simulink model "ofdm_fdm"  (Simulink 5.0)
settings: Solver=ode45  StartTime=0.0  StopTime=1  RelTol=1e-3
undefined symbols (not defined in the file): Fs
libraries: dspsrcs4 x10, dspsigops x6, commdigbbndpm2 x5, commrandsrc2 x5, dsparch4 x5, dspsnks4 x2, dspbuff3 x2, dspxfrm3 x1
settings Model: LastModifiedBy=Daiming Qu

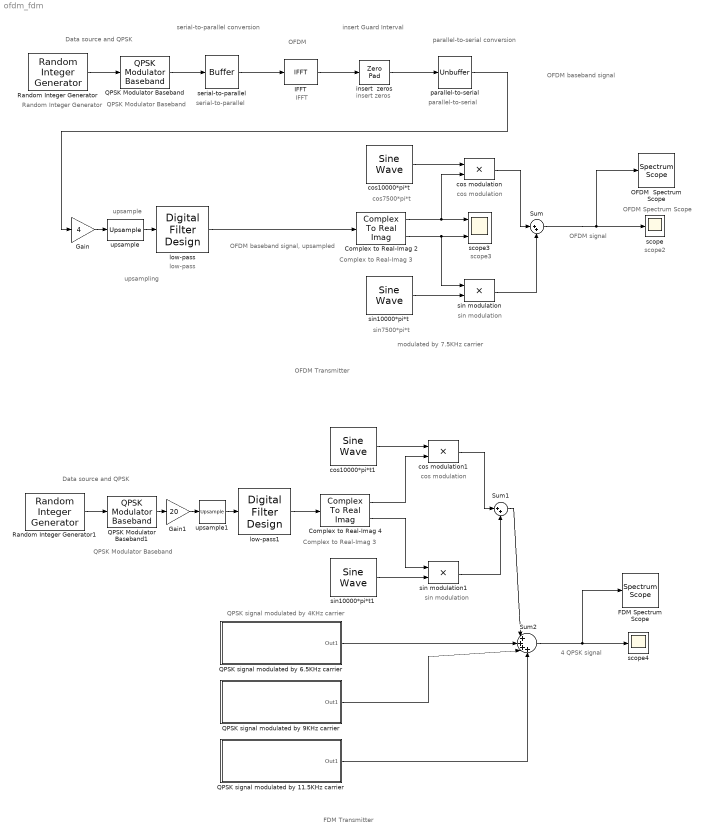
== system ofdm_fdm ==
  note: cos modulation
  note: Complex to
      | Real-Imag
      | 3
  note: Data source and QPSK
  note: QPSK
      | Modulator
      | Baseband
  note: QPSK signal modulated by 4KHz carrier
  note: sin modulation
  note: 4 QPSK signal
  note: FDM Transmitter
  note: serial-to-parallel
      |  conversion
  note: parallel-to-serial
      | conversion
  note: insert
      | Guard Interval
  note: OFDM
  note: modulated by
      | 7.5KHz carrier
  note: OFDM signal
  note: Random Integer
      | Generator
  note: QPSK
      | Modulator
      | Baseband
  note: serial-to-parallel
  note: IFFT
  note: insert
      | zeros
  note: parallel-to-serial
  note: upsample
  note: low-pass
  note: Complex to
      | Real-Imag
      | 3
  note: cos modulation
  note: sin modulation
  note: cos7500*pi*t
  note: sin7500*pi*t
  note: scope2
  note: OFDM Spectrum
      | Scope
  note: OFDM baseband signal
  note: scope3
  note: OFDM baseband
      | signal, upsampled
  note: upsampling
  note: Data source and QPSK
  note: OFDM Transmitter
  Complex to Real-Imag 2 : ComplexToRealImag
  Complex to Real-Imag 4 : ComplexToRealImag
  FDM Spectrum Scope : dspsnks4/Spectrum Scope  ScopeProperties=on  Domain=Frequency  HorizSpan=1  UseBuffer=on  BufferSize=2048  Overlap=0  inpFftLenInherit=off  FFTlength=2048  numAvg=128  DisplayProperties=off  AxisGrid=on  Memory=off  FrameNumber=on  AxisLegend=off  AxisZoom=off  OpenScopeAtSimStart=on  OpenScopeImmediately=off  FigPos=[34 274 560 420]  AxisProperties=off  XUnits=Hertz  XRange=[-Fs/2...Fs/2]  InheritXIncr=on  XIncr=1.0  XLabel=Samples  YUnits=dB  YLabel=Magnitude, dB  LineProperties=off  LineColors=[0 0 1]
      settings: YMin=-65  YMax=5
  Gain : Gain  Gain=4  SaturateOnIntegerOverflow=on
  Gain1 : Gain  Gain=20  SaturateOnIntegerOverflow=on
  IFFT : dspxfrm3/IFFT  CompMethod=Trigonometric fcn  TableOpt=Speed  BitRevOrder=off  cs_in=off  SkipNorm=on  mode=Real
  OFDM  Spectrum Scope : dspsnks4/Spectrum Scope  ScopeProperties=on  Domain=Frequency  HorizSpan=1  UseBuffer=on  BufferSize=2048  Overlap=0  inpFftLenInherit=off  FFTlength=2048  numAvg=128  DisplayProperties=off  AxisGrid=on  Memory=off  FrameNumber=on  AxisLegend=off  AxisZoom=off  OpenScopeAtSimStart=on  OpenScopeImmediately=off  FigPos=[446 60 560 420]  AxisProperties=off  XUnits=Hertz  XRange=[-Fs/2...Fs/2]  InheritXIncr=on  XIncr=1.0  XLabel=Samples  YUnits=dB  YLabel=Magnitude, dB  LineProperties=off  LineColors=[0 0 1]
      settings: YMin=-45  YMax=15
  QPSK Modulator Baseband : commdigbbndpm2/QPSK Modulator Baseband  InType=Integer  Enc=Binary  Ph=0  numSamp=1
  QPSK Modulator Baseband1 : commdigbbndpm2/QPSK Modulator Baseband  InType=Integer  Enc=Binary  Ph=0  numSamp=1
  QPSK signal modulated by 11.5KHz carrier : Subsystem
  QPSK signal modulated by 6.5KHz carrier : Subsystem
  QPSK signal modulated by 9KHz carrier : Subsystem
  Random Integer Generator : commrandsrc2/Random Integer Generator  mul=4  seed=37  Ts=1/6400  frameBased=off  sampPerFrame=1  orient=off
  Random Integer Generator1 : commrandsrc2/Random Integer Generator  mul=4  seed=37  Ts=1/1600  frameBased=off  sampPerFrame=1  orient=off
  Sum : Sum  Inputs=|++  SaturateOnIntegerOverflow=on
  Sum1 : Sum  Inputs=|++  SaturateOnIntegerOverflow=on
  Sum2 : Sum  Inputs=|++++  SaturateOnIntegerOverflow=on
  cos modulation : Product  SaturateOnIntegerOverflow=on
  cos modulation1 : Product  SaturateOnIntegerOverflow=on
  cos10000*pi*t : dspsrcs4/Sine Wave  Amplitude=1  Frequency=7500  Phase=pi/2  SampleMode=Discrete  OutComplex=Real  CompMethod=Trigonometric fcn  TableSize=Speed  SampleTime=1/32000  SamplesPerFrame=1  dataType=double  wordLen=16  udDataType=sfix(16)  fracBitsMode=Best precision  numFracBits=14  ResetState=Restart at time zero
  cos10000*pi*t1 : dspsrcs4/Sine Wave  Amplitude=1  Frequency=4000  Phase=pi/2  SampleMode=Discrete  OutComplex=Real  CompMethod=Trigonometric fcn  TableSize=Speed  SampleTime=1/32000  SamplesPerFrame=1  dataType=double  wordLen=16  udDataType=sfix(16)  fracBitsMode=Best precision  numFracBits=14  ResetState=Restart at time zero
  insert  zeros : dspsigops/Zero Pad  padSigAt=End  zpadAlong=Columns  padNumOutRowsSpecMethod=User-specified  numOutRows=80  padNumOutColsSpecMethod=User-specified  numOutCols=1  trunc_flag=None
  low-pass : dsparch4/Digital Filter Design
  low-pass1 : dsparch4/Digital Filter Design
  parallel-to-serial : dspbuff3/Unbuffer  ic=0
  scope : Scope
      settings: YMin=-0.1  YMax=0.3  SaveName=ScopeData3
  scope3 : Scope  NumInputPorts=2
      settings: YMin=-0.1~-5  YMax=0.3~5
  scope4 : Scope
      settings: YMin=-0.1  YMax=0.3
  serial-to-parallel : dspbuff3/Buffer  N=64  V=0  ic=0
  sin modulation : Product  SaturateOnIntegerOverflow=on
  sin modulation1 : Product  SaturateOnIntegerOverflow=on
  sin10000*pi*t : dspsrcs4/Sine Wave  Amplitude=1  Frequency=7500  Phase=0  SampleMode=Discrete  OutComplex=Real  CompMethod=Trigonometric fcn  TableSize=Speed  SampleTime=1/32000  SamplesPerFrame=1  dataType=double  wordLen=16  udDataType=sfix(16)  fracBitsMode=Best precision  numFracBits=14  ResetState=Restart at time zero
  sin10000*pi*t1 : dspsrcs4/Sine Wave  Amplitude=1  Frequency=4000  Phase=0  SampleMode=Discrete  OutComplex=Real  CompMethod=Trigonometric fcn  TableSize=Speed  SampleTime=1/32000  SamplesPerFrame=1  dataType=double  wordLen=16  udDataType=sfix(16)  fracBitsMode=Best precision  numFracBits=14  ResetState=Restart at time zero
  upsample : dspsigops/Upsample  N=4  phase=1  ic=0  mode=Maintain input frame size
  upsample1 : dspsigops/Upsample  N=20  phase=1  ic=0  mode=Maintain input frame size
  wires:
  low-pass1/1 -> Complex to Real-Imag 4/1
  upsample1/1 -> low-pass1/1
  cos10000*pi*t1/1 -> cos modulation1/1
  sin modulation1/1 -> Sum1/2
  cos modulation1/1 -> Sum1/1
  Complex to Real-Imag 4/2 -> sin modulation1/1
  sin10000*pi*t1/1 -> sin modulation1/2
  Complex to Real-Imag 4/1 -> cos modulation1/2
  Random Integer Generator1/1 -> QPSK Modulator Baseband1/1
  Sum1/1 -> Sum2/1
  QPSK signal modulated by 11.5KHz carrier/1(Out1) -> Sum2/4
  Sum2/1 -> FDM Spectrum Scope/1, scope4/1
  QPSK signal modulated by 6.5KHz carrier/1(Out1) -> Sum2/2
  QPSK signal modulated by 9KHz carrier/1(Out1) -> Sum2/3
  insert  zeros/1 -> parallel-to-serial/1
  low-pass/1 -> Complex to Real-Imag 2/1
  cos10000*pi*t/1 -> cos modulation/1
  Complex to Real-Imag 2/1 -> cos modulation/2, scope3/1
  sin10000*pi*t/1 -> sin modulation/2
  Complex to Real-Imag 2/2 -> sin modulation/1, scope3/2
  cos modulation/1 -> Sum/1
  sin modulation/1 -> Sum/2
  Sum/1 -> scope/1, OFDM  Spectrum Scope/1
  serial-to-parallel/1 -> IFFT/1
  IFFT/1 -> insert  zeros/1
  Random Integer Generator/1 -> QPSK Modulator Baseband/1
  QPSK Modulator Baseband/1 -> serial-to-parallel/1
  upsample/1 -> low-pass/1
  parallel-to-serial/1 -> Gain/1
  Gain/1 -> upsample/1
  QPSK Modulator Baseband1/1 -> Gain1/1
  Gain1/1 -> upsample1/1

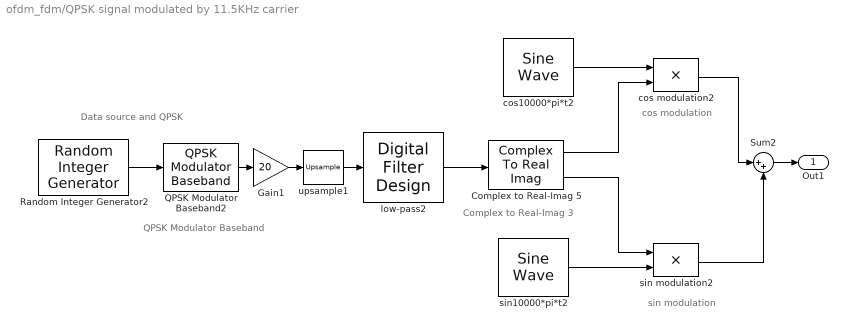
== system ofdm_fdm/QPSK signal modulated by 11.5KHz carrier ==
  note: cos modulation
  note: Complex to
      | Real-Imag
      | 3
  note: Data source and QPSK
  note: QPSK
      | Modulator
      | Baseband
  note: sin modulation
  Complex to Real-Imag 5 : ComplexToRealImag
  Gain1 : Gain  Gain=20  SaturateOnIntegerOverflow=on
  QPSK Modulator Baseband2 : commdigbbndpm2/QPSK Modulator Baseband  InType=Integer  Enc=Binary  Ph=0  numSamp=1
  Random Integer Generator2 : commrandsrc2/Random Integer Generator  mul=4  seed=15  Ts=1/1600  frameBased=off  sampPerFrame=1  orient=off
  Sum2 : Sum  Inputs=|++  SaturateOnIntegerOverflow=on
  cos modulation2 : Product  SaturateOnIntegerOverflow=on
  cos10000*pi*t2 : dspsrcs4/Sine Wave  Amplitude=1  Frequency=11500  Phase=pi/2  SampleMode=Discrete  OutComplex=Real  CompMethod=Trigonometric fcn  TableSize=Speed  SampleTime=1/32000  SamplesPerFrame=1  dataType=double  wordLen=16  udDataType=sfix(16)  fracBitsMode=Best precision  numFracBits=14  ResetState=Restart at time zero
  low-pass2 : dsparch4/Digital Filter Design
  sin modulation2 : Product  SaturateOnIntegerOverflow=on
  sin10000*pi*t2 : dspsrcs4/Sine Wave  Amplitude=1  Frequency=11500  Phase=0  SampleMode=Discrete  OutComplex=Real  CompMethod=Trigonometric fcn  TableSize=Speed  SampleTime=1/32000  SamplesPerFrame=1  dataType=double  wordLen=16  udDataType=sfix(16)  fracBitsMode=Best precision  numFracBits=14  ResetState=Restart at time zero
  upsample1 : dspsigops/Upsample  N=20  phase=1  ic=0  mode=Maintain input frame size
  Out1 : Outport
  wires:
  low-pass2/1 -> Complex to Real-Imag 5/1
  cos10000*pi*t2/1 -> cos modulation2/1
  sin modulation2/1 -> Sum2/2
  cos modulation2/1 -> Sum2/1
  Complex to Real-Imag 5/2 -> sin modulation2/1
  sin10000*pi*t2/1 -> sin modulation2/2
  Complex to Real-Imag 5/1 -> cos modulation2/2
  Random Integer Generator2/1 -> QPSK Modulator Baseband2/1
  Sum2/1 -> Out1/1
  Gain1/1 -> upsample1/1
  QPSK Modulator Baseband2/1 -> Gain1/1
  upsample1/1 -> low-pass2/1

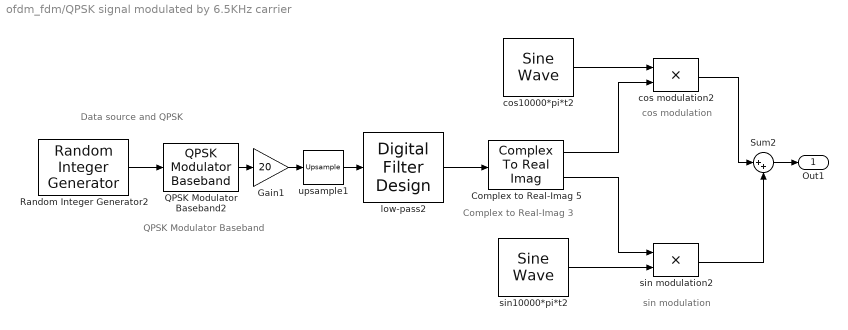
== system ofdm_fdm/QPSK signal modulated by 6.5KHz carrier ==
  note: cos modulation
  note: Complex to
      | Real-Imag
      | 3
  note: Data source and QPSK
  note: QPSK
      | Modulator
      | Baseband
  note: sin modulation
  Complex to Real-Imag 5 : ComplexToRealImag
  Gain1 : Gain  Gain=20  SaturateOnIntegerOverflow=on
  QPSK Modulator Baseband2 : commdigbbndpm2/QPSK Modulator Baseband  InType=Integer  Enc=Binary  Ph=0  numSamp=1
  Random Integer Generator2 : commrandsrc2/Random Integer Generator  mul=4  seed=76  Ts=1/1600  frameBased=off  sampPerFrame=1  orient=off
  Sum2 : Sum  Inputs=|++  SaturateOnIntegerOverflow=on
  cos modulation2 : Product  SaturateOnIntegerOverflow=on
  cos10000*pi*t2 : dspsrcs4/Sine Wave  Amplitude=1  Frequency=6500  Phase=pi/2  SampleMode=Discrete  OutComplex=Real  CompMethod=Trigonometric fcn  TableSize=Speed  SampleTime=1/32000  SamplesPerFrame=1  dataType=double  wordLen=16  udDataType=sfix(16)  fracBitsMode=Best precision  numFracBits=14  ResetState=Restart at time zero
  low-pass2 : dsparch4/Digital Filter Design
  sin modulation2 : Product  SaturateOnIntegerOverflow=on
  sin10000*pi*t2 : dspsrcs4/Sine Wave  Amplitude=1  Frequency=6500  Phase=0  SampleMode=Discrete  OutComplex=Real  CompMethod=Trigonometric fcn  TableSize=Speed  SampleTime=1/32000  SamplesPerFrame=1  dataType=double  wordLen=16  udDataType=sfix(16)  fracBitsMode=Best precision  numFracBits=14  ResetState=Restart at time zero
  upsample1 : dspsigops/Upsample  N=20  phase=1  ic=0  mode=Maintain input frame size
  Out1 : Outport
  wires:
  low-pass2/1 -> Complex to Real-Imag 5/1
  cos10000*pi*t2/1 -> cos modulation2/1
  sin modulation2/1 -> Sum2/2
  cos modulation2/1 -> Sum2/1
  Complex to Real-Imag 5/2 -> sin modulation2/1
  sin10000*pi*t2/1 -> sin modulation2/2
  Complex to Real-Imag 5/1 -> cos modulation2/2
  Random Integer Generator2/1 -> QPSK Modulator Baseband2/1
  Sum2/1 -> Out1/1
  Gain1/1 -> upsample1/1
  QPSK Modulator Baseband2/1 -> Gain1/1
  upsample1/1 -> low-pass2/1

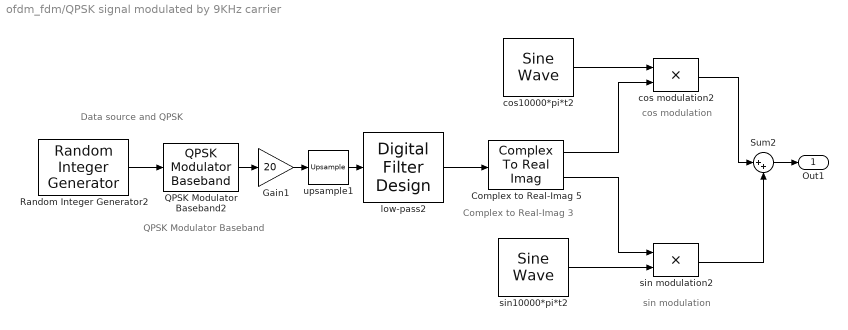
== system ofdm_fdm/QPSK signal modulated by 9KHz carrier ==
  note: cos modulation
  note: Complex to
      | Real-Imag
      | 3
  note: Data source and QPSK
  note: QPSK
      | Modulator
      | Baseband
  note: sin modulation
  Complex to Real-Imag 5 : ComplexToRealImag
  Gain1 : Gain  Gain=20  SaturateOnIntegerOverflow=on
  QPSK Modulator Baseband2 : commdigbbndpm2/QPSK Modulator Baseband  InType=Integer  Enc=Binary  Ph=0  numSamp=1
  Random Integer Generator2 : commrandsrc2/Random Integer Generator  mul=4  seed=21  Ts=1/1600  frameBased=off  sampPerFrame=1  orient=off
  Sum2 : Sum  Inputs=|++  SaturateOnIntegerOverflow=on
  cos modulation2 : Product  SaturateOnIntegerOverflow=on
  cos10000*pi*t2 : dspsrcs4/Sine Wave  Amplitude=1  Frequency=9000  Phase=pi/2  SampleMode=Discrete  OutComplex=Real  CompMethod=Trigonometric fcn  TableSize=Speed  SampleTime=1/32000  SamplesPerFrame=1  dataType=double  wordLen=16  udDataType=sfix(16)  fracBitsMode=Best precision  numFracBits=14  ResetState=Restart at time zero
  low-pass2 : dsparch4/Digital Filter Design
  sin modulation2 : Product  SaturateOnIntegerOverflow=on
  sin10000*pi*t2 : dspsrcs4/Sine Wave  Amplitude=1  Frequency=9000  Phase=0  SampleMode=Discrete  OutComplex=Real  CompMethod=Trigonometric fcn  TableSize=Speed  SampleTime=1/32000  SamplesPerFrame=1  dataType=double  wordLen=16  udDataType=sfix(16)  fracBitsMode=Best precision  numFracBits=14  ResetState=Restart at time zero
  upsample1 : dspsigops/Upsample  N=20  phase=1  ic=0  mode=Maintain input frame size
  Out1 : Outport
  wires:
  low-pass2/1 -> Complex to Real-Imag 5/1
  cos10000*pi*t2/1 -> cos modulation2/1
  sin modulation2/1 -> Sum2/2
  cos modulation2/1 -> Sum2/1
  Complex to Real-Imag 5/2 -> sin modulation2/1
  sin10000*pi*t2/1 -> sin modulation2/2
  Complex to Real-Imag 5/1 -> cos modulation2/2
  Random Integer Generator2/1 -> QPSK Modulator Baseband2/1
  Sum2/1 -> Out1/1
  Gain1/1 -> upsample1/1
  QPSK Modulator Baseband2/1 -> Gain1/1
  upsample1/1 -> low-pass2/1
